simulink model "AHRSv2"  (R2021a)
settings: Solver=FixedStepAuto  StartTime=0.0  StopTime=inf  FixedStep=0.01  RelTol=1e-3
undefined symbols (not defined in the file or in its folder): sigbuilder_block
settings Model: EnablePacing=on  Creator=kubab  LastModifiedBy=kubab

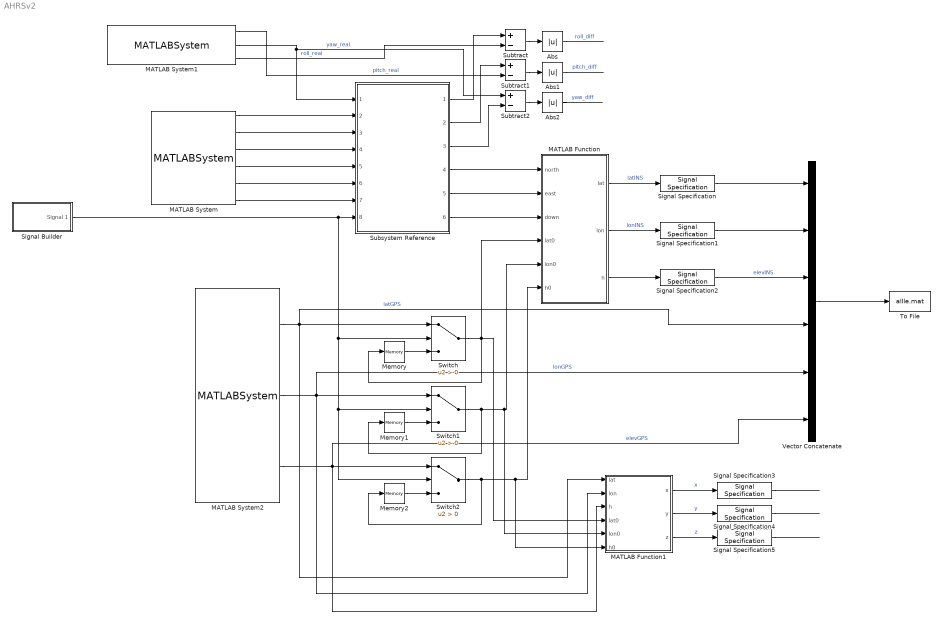
== system AHRSv2 ==
  Abs : Abs
  Abs1 : Abs
  Abs2 : Abs
  MATLAB Function : MATLAB Function  TreatAsAtomicUnit=on
  MATLAB Function1 : MATLAB Function  TreatAsAtomicUnit=on
  MATLAB System : MATLABSystem  System=IMU  SimulateUsing=Code generation
      mask Type: IMU
      mask Display:
      | disp('IMU');
      | port_label('output',1,'p');
      | port_label('output',2,'q');
      | port_label('output',3,'r');
      | port_label('output',4,'axial_acceleration');
      | port_label('output',5,'normal_acceleration');
      | port_label('output',6,'side_acceleration');
  MATLAB System1 : MATLABSystem  System=Angles_real  SimulateUsing=Code generation
      mask Type: Angles_real
      mask Display:
      | disp('Angles_real');
      | port_label('output',1,'pitch');
      | port_label('output',2,'true_heading');
      | port_label('output',3,'roll');
  MATLAB System2 : MATLABSystem  System=GPS  SimulateUsing=Code generation
      mask Type: GPS
      mask Display:
      | disp('GPS');
      | port_label('output',1,'lat');
      | port_label('output',2,'lon');
      | port_label('output',3,'elevation');
  Memory : Memory
  Memory1 : Memory
  Memory2 : Memory
  Signal Builder : Subsystem  Tag=STV Subsys  LoadFcn=sigbuilder_block('load');  StartFcn=sigbuilder_block('start');  StopFcn=sigbuilder_block('stop');  ClipboardFcn=sigbuilder_block('clipboard');  mask(Sigbuilder block){tuvar=[0:10]}
      mask help: Simulink:masks:SigbuilderBlock_MD
      mask init:
      | if ~strcmp(get_param(bdroot(gcbh),'SimulationStatus'),'stopped') tuvar = sigbuilder_block('maskInit'); end
      settings: CopyFcn=sigbuilder_block('copy');  DeleteFcn=sigbuilder_block('delete');  ModelCloseFcn=sigbuilder_block('modelClose');  PreSaveFcn=sigbuilder_block('preSave');  PauseFcn=sigbuilder_block('pause');  ContinueFcn=sigbuilder_block('continue');  NameChangeFcn=sigbuilder_block('namechange');  OpenFcn=sigbuilder_block('open',[437.6 199.2 550.4 400 ]);  CloseFcn=sigbuilder_block('close');
      mask Display: plot(0, 0, 100, 100,[2, 2, 32, 32, 2], [68, 8, 8, 68, 68],[32, 2], [38, 38], [32, 19, 2],[53, 60, 44], [32, 17, 17, 2],[16, 16, 31, 31]);txt = getActiveGroup(gcbh);text(2, 100, txt,'verticalAlignment', 'top');
  Signal Specification{,1..5} (6 alike) : SignalSpecification  OutDataTypeStr=double  Dimensions=1
  Subsystem Reference : Subsystem  ReferencedSubsystem=INS_subs
  Subtract : Sum  Inputs=+-
  Subtract1 : Sum  Inputs=+-
  Subtract2 : Sum  Inputs=+-
  Switch : Switch  Criteria=u2 > Threshold
  Switch1 : Switch  Criteria=u2 > Threshold
  Switch2 : Switch  Criteria=u2 > Threshold
  To File : ToFile  Filename=allle.mat  MatrixName=coordinates  SampleTime=0.12
  Vector Concatenate : Concatenate  NumInputs=6
  wires:
  MATLAB System/1 -> Subsystem Reference/2
  MATLAB System/2 -> Subsystem Reference/3
  MATLAB System/3 -> Subsystem Reference/4
  MATLAB System/4 -> Subsystem Reference/5
  MATLAB System/5 -> Subsystem Reference/6
  MATLAB System/6 -> Subsystem Reference/7
  Signal Builder/1(Signal 1) -> Switch2/2, Switch1/2, Switch/2, Subsystem Reference/8
  MATLAB System1/2 -> Subtract2/1, Subsystem Reference/1  "yaw_real"
  MATLAB Function/1(lat) -> Signal Specification/1  "latINS"
  MATLAB Function/2(lon) -> Signal Specification1/1  "lonINS"
  MATLAB Function/3(h) -> Signal Specification2/1
  Vector Concatenate/1 -> To File/1
  Subsystem Reference/4 -> MATLAB Function/1(north)
  Subsystem Reference/5 -> MATLAB Function/2(east)
  Subsystem Reference/6 -> MATLAB Function/3(down)
  Memory/1 -> Switch/3
  Memory1/1 -> Switch1/3
  Memory2/1 -> Switch2/3
  Signal Specification/1 -> Vector Concatenate/1
  Signal Specification1/1 -> Vector Concatenate/2
  Signal Specification2/1 -> Vector Concatenate/3  "elevINS"
  Subsystem Reference/1 -> Subtract/1
  MATLAB System1/3 -> Subtract/2  "roll_real"
  Subtract/1 -> Abs/1
  Abs/1 -> ?  "roll_diff"
  MATLAB System1/1 -> Subtract1/2  "pitch_real"
  Subtract1/1 -> Abs1/1
  Abs1/1 -> ?  "pitch_diff"
  Subsystem Reference/2 -> Subtract1/1
  Subtract2/1 -> Abs2/1
  Abs2/1 -> ?  "yaw_diff"
  Subsystem Reference/3 -> Subtract2/2
  Signal Specification3/1 -> ?
  Signal Specification5/1 -> ?
  Signal Specification4/1 -> ?
  MATLAB System2/2 -> MATLAB Function1/2(lon), Vector Concatenate/5, Switch1/1  "lonGPS"
  MATLAB Function1/1(x) -> Signal Specification3/1  "x"
  MATLAB Function1/2(y) -> Signal Specification4/1  "y"
  Switch1/1 -> MATLAB Function1/5(lon0), MATLAB Function/5(lon0), Memory1/1
  MATLAB System2/3 -> MATLAB Function1/3(h), Vector Concatenate/6, Switch2/1  "elevGPS"
  Switch/1 -> MATLAB Function1/4(lat0), MATLAB Function/4(lat0), Memory/1
  Switch2/1 -> Memory2/1, MATLAB Function1/6(h0), MATLAB Function/6(h0)
  MATLAB Function1/3(z) -> Signal Specification5/1  "z"
  MATLAB System2/1 -> MATLAB Function1/1(lat), Switch/1, Vector Concatenate/4  "latGPS"

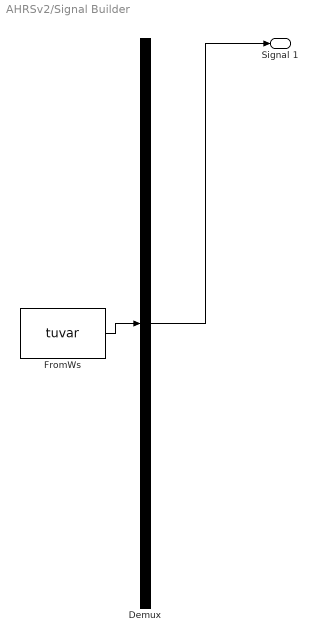
== system AHRSv2/Signal Builder ==
  Demux : Demux  Tag=STV Demux  Outputs=1
      settings: DisplayOption=none
  FromWs : FromWorkspace  Tag=STV FromWs  VariableName=tuvar
      SigBuilderData=|
      | common.afterFinalStr = 'Extrapolate'
      | common.sampleTime = 0
      | dataSet.timeRange = [0 10]
      | dataSet.name = 'Group 1'
      | sbobj.Groups.Name = 'Group 1'
      | sbobj.Groups.Signals.Name = 'Signal 1'
      | sbobj.Groups.Signals.XData = [0 5.02 5.02 10]
      | sbobj.Groups.Signals.YData = [1 1 0 0]
  Signal 1 : Outport  Tag=STV Outport
  wires:
  Demux/1 -> Signal 1/1
  FromWs/1 -> Demux/1

== matlab function AHRSv2/MATLAB Function ==
  data: north input; lat output; east input; down input; lat0 input; lon0 input; h0 input; lon output; h output
function [lat,lon,h] = ned2geo(north, east, down, lat0, lon0, h0)

[xlat, xlon, xh] = ned2geodetic(north, east, down, lat0, lon0, h0, wgs84Ellipsoid);

lat = xlat;
lon = xlon;
h = xh;

== matlab function AHRSv2/MATLAB Function1 ==
  data: x output; lat input; y output; lon input; h input; lat0 input; lon0 input; h0 input; z output
function [x,y,z] = geo2ned(lat, lon, h, lat0, lon0, h0)
[n,e,d] = geodetic2ned(lat,lon,h,lat0,lon0,h0,wgs84Ellipsoid);
x = n;
y = e;
z = d;
